simulink library "quat_mul"  (R2023b)
settings: Solver=VariableStepAuto  StartTime=0.0  StopTime=10.0  RelTol=1e-3
settings Model: Creator=robin  LastModifiedBy=robin

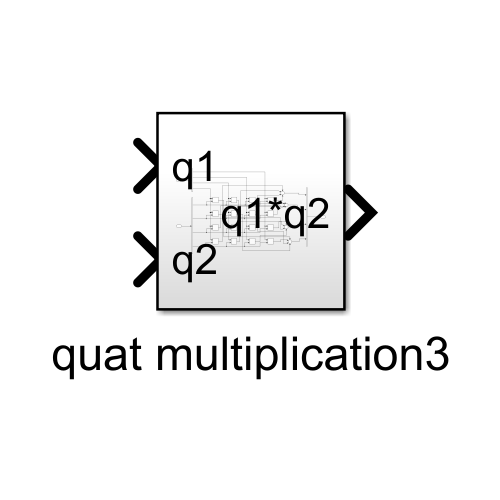
[thumbnail: Simulink's stored preview of the top-level diagram]
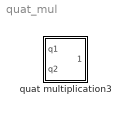
== system quat_mul ==
  quat multiplication3 : Subsystem

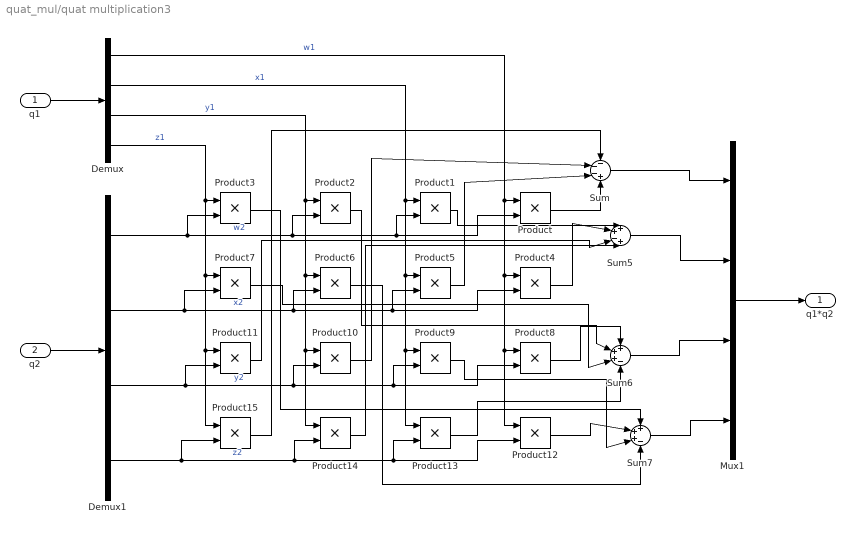
== system quat_mul/quat multiplication3 ==
  q1 : Inport
  q2 : Inport  Port=2
  Demux : Demux
  Demux1 : Demux
  Mux1 : Mux
  Product{,1..15} (16 alike) : Product
  Sum : Sum  Inputs=---+
  Sum5 : Sum  Inputs=++-+
  Sum6 : Sum  Inputs=+++-
  Sum7 : Sum  Inputs=+++-
  q1*q2 : Outport
  wires:
  Sum5/1 -> Mux1/2
  Product/1 -> Sum/4
  Product9/1 -> Sum7/3
  Demux/1 -> Product12/1, Product8/1, Product4/1, Product/1  "w1"
  Demux1/3 -> Product8/2, Product9/2, Product10/2, Product11/2  "y2"
  Demux/2 -> Product13/1, Product9/1, Product5/1, Product1/1  "x1"
  Product6/1 -> Sum7/4
  Product4/1 -> Sum5/2
  Demux1/1 -> Product/2, Product1/2, Product2/2, Product3/2  "w2"
  Sum/1 -> Mux1/1
  Product3/1 -> Sum7/1
  Product15/1 -> Sum/1
  Product1/1 -> Sum5/1
  Product2/1 -> Sum6/2
  Demux/4 -> Product15/1, Product11/1, Product7/1, Product3/1  "z1"
  Sum6/1 -> Mux1/3
  Demux1/2 -> Product4/2, Product5/2, Product6/2, Product7/2  "x2"
  Demux1/4 -> Product12/2, Product13/2, Product14/2, Product15/2  "z2"
  Product14/1 -> Sum5/4
  Mux1/1 -> q1*q2/1
  Sum7/1 -> Mux1/4
  Demux/3 -> Product14/1, Product10/1, Product6/1, Product2/1  "y1"
  Product13/1 -> Sum6/4
  Product8/1 -> Sum6/1
  q2/1 -> Demux1/1
  q1/1 -> Demux/1
  Product11/1 -> Sum5/3
  Product7/1 -> Sum6/3
  Product10/1 -> Sum/2
  Product5/1 -> Sum/3
  Product12/1 -> Sum7/2
